simulink model "openloop_sys"  (R2018b)
settings: Solver=VariableStepAuto  StartTime=0.0  StopTime=300000  RelTol=1e-3
values from neighbouring files (symbols this model uses):
  Lat1_den = [1, 4.641e-5, 0.0002839]    [ControlSystem.m]
  Lat1_num = [0.00835, 0.001745]    [ControlSystem.m]
  Lat2_den = [1, 0.4456, 27.55, 4.316]    [ControlSystem.m]
  Lat2_num = [0.0002557, -0.02031, 0.05613]    [ControlSystem.m]
  Lon_den = [1,0.3537, 0.1394,0.002024]    [ControlSystem.m]
  Lon_num = [2.423, 0.1097]    [ControlSystem.m]
settings Model: Creator=nmass  LastModifiedBy=nmass

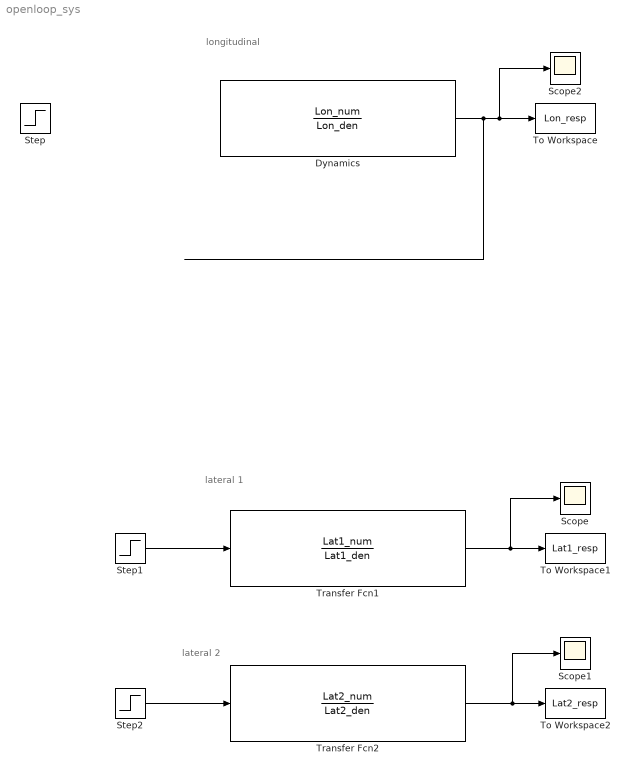
== system openloop_sys ==
  note: lateral 2
  note: lateral 1
  note: longitudinal
  Dynamics : TransferFcn  Numerator=Lon_num  Denominator=Lon_den  ContinuousStateAttributes="\"Longitudinal\""
  Scope : Scope
  Scope1 : Scope
  Scope2 : Scope
  Step : Step  SampleTime=0
  Step1 : Step  SampleTime=0
  Step2 : Step  SampleTime=0
  To Workspace : ToWorkspace  VariableName=Lon_resp  SaveFormat=Timeseries  SampleTime=-1
  To Workspace1 : ToWorkspace  VariableName=Lat1_resp  SaveFormat=Timeseries  SampleTime=-1
  To Workspace2 : ToWorkspace  VariableName=Lat2_resp  SaveFormat=Timeseries  SampleTime=-1
  Transfer Fcn1 : TransferFcn  Numerator=Lat1_num  Denominator=Lat1_den  ContinuousStateAttributes="\"Longitudinal\""
  Transfer Fcn2 : TransferFcn  Numerator=Lat2_num  Denominator=Lat2_den  ContinuousStateAttributes="\"Longitudinal\""
  wires:
  Dynamics/1 -> Scope2/1, To Workspace/1
  Step1/1 -> Transfer Fcn1/1
  Step2/1 -> Transfer Fcn2/1
  Transfer Fcn1/1 -> Scope/1, To Workspace1/1
  Transfer Fcn2/1 -> Scope1/1, To Workspace2/1
